simulink model "rendezvous_optimization_GWO"  (R2023a)
settings: Solver=VariableStepAuto  StartTime=0.0  StopTime=100  RelTol=1e-3
undefined symbols (not defined in the file): Ax, Ax_i, Ay, Ay_i, Az, Bx, Bx_i, By, By_i, Bz, Cx, Cx_i, Cy, Cy_i, Cz, IC_x_init, IC_y_init, juliandate, m0, mDot, OC_x_init, OC_y_init, OC_z_init, omega_T, Ve
(part 2 of 2)

== matlab function rendezvous_optimization_GWO/Deputy Spacecraft/Guidance and Control/Control/Translational Controller/Inner Controller-x/Subsystem/MATLAB Function ==
  settings: updateMethod=DISCRETE
  data: bestKi output; bestKp output; bestKd output; error input
function [bestKi,bestKp,bestKd] = grey_wolf(error)
% tuneAndSimulate.m
%----------------------------------------------------------------------
% This script loads your state-space plant, runs the Grey Wolf Optimizer
% to tune PID gains offline, injects those gains into your Simulink model,
% and then runs the simulation.
%
% USAGE:
% 1) Edit the “Define plant” section to load or assign A, B, C, D.
% 2) Set your Simulink model name and PID block path.
% 3) Run this script.
%----------------------------------------------------------------------

%% 1) Define or load your state-space plant matrices
%sys = ss(Ax,Bx,Cx,Dx);

%% 2) GWO parameters for PID tuning
numWolves = 100;       % population size
maxIter   = 100;      % iterations
lb        = [0   0   0];    % [Kp_min, Ki_min, Kd_min]
ub        = [10 5 10];    % [Kp_max, Ki_max, Kd_max]

% Run Grey Wolf Optimizer
bestGains = runGWO(numWolves, maxIter, lb, ub);
bestKp   = bestGains(1);
bestKi   = bestGains(2);
bestKd   = bestGains(3);
%fprintf('Optimized gains: Kp=%.4f, Ki=%.4f, Kd=%.4f\n', bestKp, bestKi, bestKd);

%======================================================================
% Local function: runGWO
%======================================================================
function bestGains = runGWO(numWolves, maxIter, lb, ub)
    dim = 3;  % tuning [Kp, Ki, Kd]
    % Initialize wolves
    pos = rand(numWolves,dim) .* (ub - lb) + lb;
    alpha_pos = zeros(1,dim);    alpha_score = inf;
    beta_pos  = zeros(1,dim);    beta_score  = inf;
    delta_pos = zeros(1,dim);    delta_score = inf;

    % Main GWO loop
    for iter = 1:maxIter
        for i = 1:numWolves
            score = error;
            if score < alpha_score
                delta_score = beta_score;   delta_pos = beta_pos;
                beta_score  = alpha_score;  beta_pos  = alpha_pos;
                alpha_score = score;        alpha_pos = pos(i,:);
            elseif score < beta_score
                delta_score = beta_score;   delta_pos = beta_pos;
                beta_score  = score;        beta_pos  = pos(i,:);
            elseif score < delta_score
                delta_score = score;        delta_pos = pos(i,:);
            end
        end
        a = 2 * (1 - iter/maxIter);
        for i = 1:numWolves
            for j = 1:dim
                r1 = rand; r2 = rand;
                A1 = 2*a*r1 - a; C1 = 2*r2;
                D_alpha = abs(C1*alpha_pos(j) - pos(i,j));
                X1 = alpha_pos(j) - A1*D_alpha;

                r1 = rand; r2 = rand;
                A2 = 2*a*r1 - a; C2 = 2*r2;
                D_beta  = abs(C2*beta_pos(j) - pos(i,j));
                X2 = beta_pos(j)  - A2*D_beta;

                r1 = rand; r2 = rand;
                A3 = 2*a*r1 - a; C3 = 2*r2;
                D_delta = abs(C3*delta_pos(j) - pos(i,j));
                X3 = delta_pos(j) - A3*D_delta;

                pos(i,j) = (X1 + X2 + X3)/3;
            end
            % enforce bounds
            pos(i,:) = max(min(pos(i,:), ub), lb);
        end
    end
    bestGains = alpha_pos;
end
  
end

== matlab function rendezvous_optimization_GWO/Deputy Spacecraft/Guidance and Control/Control/Translational Controller/Inner Controller-y/Subsystem/MATLAB Function ==
  settings: updateMethod=DISCRETE
  data: bestKi output; bestKp output; bestKd output; error input
function [bestKi,bestKp,bestKd] = grey_wolf(error)
% tuneAndSimulate.m
%----------------------------------------------------------------------
% This script loads your state-space plant, runs the Grey Wolf Optimizer
% to tune PID gains offline, injects those gains into your Simulink model,
% and then runs the simulation.
%
% USAGE:
% 1) Edit the “Define plant” section to load or assign A, B, C, D.
% 2) Set your Simulink model name and PID block path.
% 3) Run this script.
%----------------------------------------------------------------------

%% 1) Define or load your state-space plant matrices
%sys = ss(Ax,Bx,Cx,Dx);

%% 2) GWO parameters for PID tuning
numWolves = 100;       % population size
maxIter   = 100;      % iterations
lb        = [0   0   0];    % [Kp_min, Ki_min, Kd_min]
ub        = [10 5 10];    % [Kp_max, Ki_max, Kd_max]

% Run Grey Wolf Optimizer
bestGains = runGWO(numWolves, maxIter, lb, ub);
bestKp   = bestGains(1);
bestKi   = bestGains(2);
bestKd   = bestGains(3);
%fprintf('Optimized gains: Kp=%.4f, Ki=%.4f, Kd=%.4f\n', bestKp, bestKi, bestKd);

%======================================================================
% Local function: runGWO
%======================================================================
function bestGains = runGWO(numWolves, maxIter, lb, ub)
    dim = 3;  % tuning [Kp, Ki, Kd]
    % Initialize wolves
    pos = rand(numWolves,dim) .* (ub - lb) + lb;
    alpha_pos = zeros(1,dim);    alpha_score = inf;
    beta_pos  = zeros(1,dim);    beta_score  = inf;
    delta_pos = zeros(1,dim);    delta_score = inf;

    % Main GWO loop
    for iter = 1:maxIter
        for i = 1:numWolves
            score = error;
            if score < alpha_score
                delta_score = beta_score;   delta_pos = beta_pos;
                beta_score  = alpha_score;  beta_pos  = alpha_pos;
                alpha_score = score;        alpha_pos = pos(i,:);
            elseif score < beta_score
                delta_score = beta_score;   delta_pos = beta_pos;
                beta_score  = score;        beta_pos  = pos(i,:);
            elseif score < delta_score
                delta_score = score;        delta_pos = pos(i,:);
            end
        end
        a = 2 * (1 - iter/maxIter);
        for i = 1:numWolves
            for j = 1:dim
                r1 = rand; r2 = rand;
                A1 = 2*a*r1 - a; C1 = 2*r2;
                D_alpha = abs(C1*alpha_pos(j) - pos(i,j));
                X1 = alpha_pos(j) - A1*D_alpha;

                r1 = rand; r2 = rand;
                A2 = 2*a*r1 - a; C2 = 2*r2;
                D_beta  = abs(C2*beta_pos(j) - pos(i,j));
                X2 = beta_pos(j)  - A2*D_beta;

                r1 = rand; r2 = rand;
                A3 = 2*a*r1 - a; C3 = 2*r2;
                D_delta = abs(C3*delta_pos(j) - pos(i,j));
                X3 = delta_pos(j) - A3*D_delta;

                pos(i,j) = (X1 + X2 + X3)/3;
            end
            % enforce bounds
            pos(i,:) = max(min(pos(i,:), ub), lb);
        end
    end
    bestGains = alpha_pos;
end
  
end

== matlab function rendezvous_optimization_GWO/Deputy Spacecraft/Guidance and Control/Control/Translational Controller/Inner Controller-z/Subsystem/MATLAB Function ==
  settings: updateMethod=DISCRETE
  data: bestKi output; bestKp output; bestKd output; error input
function [bestKi,bestKp,bestKd] = grey_wolf(error)
% tuneAndSimulate.m
%----------------------------------------------------------------------
% This script loads your state-space plant, runs the Grey Wolf Optimizer
% to tune PID gains offline, injects those gains into your Simulink model,
% and then runs the simulation.
%
% USAGE:
% 1) Edit the “Define plant” section to load or assign A, B, C, D.
% 2) Set your Simulink model name and PID block path.
% 3) Run this script.
%----------------------------------------------------------------------

%% 1) Define or load your state-space plant matrices
%sys = ss(Ax,Bx,Cx,Dx);

%% 2) GWO parameters for PID tuning
numWolves = 100;       % population size
maxIter   = 100;      % iterations
lb        = [0   0   0];    % [Kp_min, Ki_min, Kd_min]
ub        = [10 5 10];    % [Kp_max, Ki_max, Kd_max]


% Run Grey Wolf Optimizer
bestGains = runGWO(numWolves, maxIter, lb, ub);
bestKp   = bestGains(1);
bestKi   = bestGains(2);
bestKd   = bestGains(3);
%fprintf('Optimized gains: Kp=%.4f, Ki=%.4f, Kd=%.4f\n', bestKp, bestKi, bestKd);

%======================================================================
% Local function: runGWO
%======================================================================
function bestGains = runGWO(numWolves, maxIter, lb, ub)
    dim = 3;  % tuning [Kp, Ki, Kd]
    % Initialize wolves
    pos = rand(numWolves,dim) .* (ub - lb) + lb;
    alpha_pos = zeros(1,dim);    alpha_score = inf;
    beta_pos  = zeros(1,dim);    beta_score  = inf;
    delta_pos = zeros(1,dim);    delta_score = inf;

    % Main GWO loop
    for iter = 1:maxIter
        for i = 1:numWolves
            score = error;
            if score < alpha_score
                delta_score = beta_score;   delta_pos = beta_pos;
                beta_score  = alpha_score;  beta_pos  = alpha_pos;
                alpha_score = score;        alpha_pos = pos(i,:);
            elseif score < beta_score
                delta_score = beta_score;   delta_pos = beta_pos;
                beta_score  = score;        beta_pos  = pos(i,:);
            elseif score < delta_score
                delta_score = score;        delta_pos = pos(i,:);
            end
        end
        a = 2 * (1 - iter/maxIter);
        for i = 1:numWolves
            for j = 1:dim
                r1 = rand; r2 = rand;
                A1 = 2*a*r1 - a; C1 = 2*r2;
                D_alpha = abs(C1*alpha_pos(j) - pos(i,j));
                X1 = alpha_pos(j) - A1*D_alpha;

                r1 = rand; r2 = rand;
                A2 = 2*a*r1 - a; C2 = 2*r2;
                D_beta  = abs(C2*beta_pos(j) - pos(i,j));
                X2 = beta_pos(j)  - A2*D_beta;

                r1 = rand; r2 = rand;
                A3 = 2*a*r1 - a; C3 = 2*r2;
                D_delta = abs(C3*delta_pos(j) - pos(i,j));
                X3 = delta_pos(j) - A3*D_delta;

                pos(i,j) = (X1 + X2 + X3)/3;
            end
            % enforce bounds
            pos(i,:) = max(min(pos(i,:), ub), lb);
        end
    end
    bestGains = alpha_pos;
end
  
end

== matlab function rendezvous_optimization_GWO/Deputy Spacecraft/Guidance and Control/Control/Translational Controller/Outer Controller-x/Controller-1/MATLAB Function1 ==
  settings: updateMethod=DISCRETE
  data: reset input; error_percent output; error input
function error_percent = error_percentage(reset,error)
% Compute gain based on percentage error using 1D look-up style logic
%
% Inputs:
%   r_des     : 3x1 desired position vector
%   r_current : 3x1 current position vector (from chaser)
%   r_init    : 3x1 initial position vector
%
% Output:
%   gain      : scalar scheduled gain

    persistent max_error;

    if reset || isempty(max_error)
        max_error = norm(error);  % store initial max error
    end
    
    e_now = norm(error);       % current error
    error_percent = (e_now / max_error)*100;       % normalized error: [0, 1]

   
end
